simulink model "Main_A"  (R2021a)
settings: Solver=daessc  StartTime=0.0  StopTime=20  RelTol=1e-3
model workspace (MAT data in the model file):
  VEH.Mass = 1181
  VEH.StaticNormalFrontLoad.FR = 264.666666667
  VEH.StaticNormalFrontLoad.FL = 264.666666667
  VEH.StaticNormalRearLoad.RR = 322
  VEH.StaticNormalRearLoad.RL = 322
  VEH.WheelBase = 3.075
  VEH.FrontAxlePositionfromCG = 1.515
  VEH.RearAxlePositionfromCG = 1.504
  VEH.HeightCG = 0.134
  VEH.FrontalArea = 2.11
  VEH.DragCoefficient = 0.33
  VEH.NumberOfWheelsPerAxle = 2
  VEH.PitchMomentInertia = 1922.66666667
  VEH.RollMomentInertia = 432.333333333
  VEH.YawMomentInertia = 2066
  VEH.SteeringRatio = 18
  VEH.TrackWidth = 1.922
  VEH.SprungMass = 1096.72266667
  VEH.InitialLongPosition = -118
  VEH.InitialLatPosition = 3.125
  VEH.InitialVertPosition = 0
  VEH.InitialRollAngle = 0
  VEH.InitialPitchAngle = 0
  VEH.InitialYawAngle = 0
  VEH.InitialLongVel = 0
  VEH.InitialLatVel = 0
  VEH.InitialVertVel = 0
  VEH.InitialRollRate = 0
  VEH.InitialPitchRate = 0
  VEH.InitialYawRate = 0
undefined symbols (not defined in the file): dT, Mu, MuSplit, P_ABSPressureRateMax, P_BrakePressureMax, P_PedalTravelRateMax, P_RefLine4SplitMue, P_RefLine_On, P_RefLineIsX, P_SplitMu_On, P_SplitMuOnlyAtBraking, P_SteeringMax, P_TorqueMax, t_Brake
libraries: sim3dlib x2, simulink_extras x1, vehdynlibsteering x1, sim3dautolib x1, simulink x1, vehdynlibviscommon x1
(part 1 of 2)
settings Model: OrderedModelArguments=off  Creator=Farid  LastModifiedBy=aguil
settings SolverCC: AlgebraicLoopSolver=TrustRegion
settings DebuggingCC: SFMachineParentedDataDiag=warning

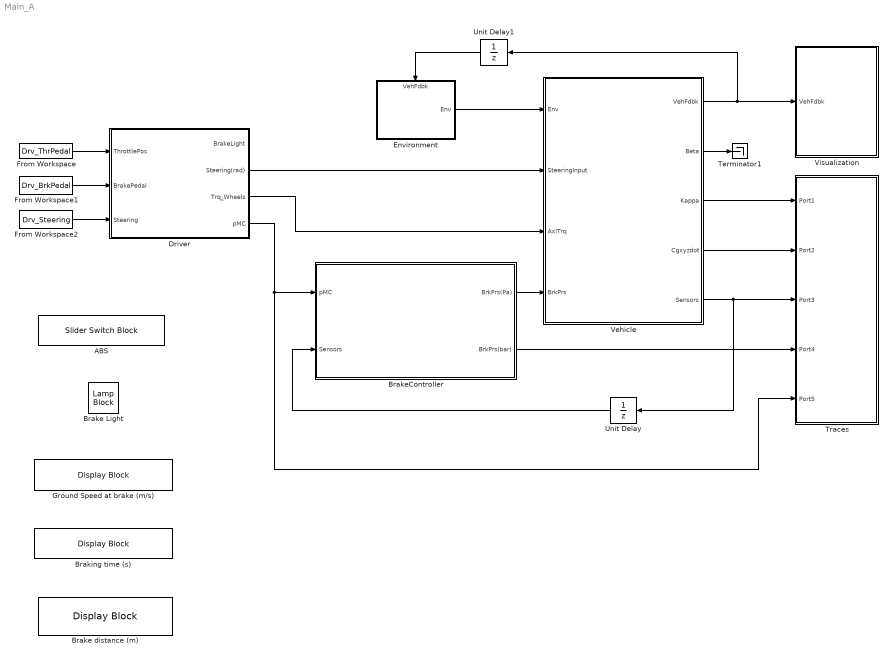
== system Main_A ==
  ABS : SliderSwitchBlock  LabelPosition=Hide
      settings: Values={{'Off', 'On'}, [0 1]}
  Brake Light : LampBlock  LabelPosition=Hide
  Brake distance (m) : DisplayBlock  LabelPosition=Hide  Format=short  Transparency=1
  BrakeController : Subsystem
      mask Display: image('ESP.jpg'); % Use "Edit Image" on toolstrip to change.
  Braking time (s) : DisplayBlock  LabelPosition=Hide  Format=short  Transparency=1
  Driver : Subsystem
  Environment : Subsystem
      settings: PortSchema="{\"entries\":[{\"content\":{\"sides\":[{\"content\":{\"connectorIds\":[]},\"type\":\"ConnectorPlacement.EquallySpacedRectSide\",\"uuid\":\"db779631-5d12-4b7d-908c-0777e0f771c7\"},{\"content\":{\"connectorIds\":[\"Out1\"],\"side\":\"RIGHT\"},\"type\":\"ConnectorPlacement.EquallySpacedRectSide\",\"uuid\":\"a6ec5440-a008-4eb7-8ac9-30b9ee520514\"},{\"content\":{\"connectorIds\":[\"In1\"],\"side\":\"TOP\"},\"type\":\"ConnectorPlacement.EquallySpacedRectSide\",\"uuid\":\"a69fe3ec-df71-47d6-bb93-a6977ac564e9\"},{\"content\":{\"connectorIds\":[],\"side\":\"HIDDEN\"},\"type\":\"ConnectorPlacement.EquallySpacedRectSide\",\"uuid\":\"922b3558-1bf2-4b3b-9005-bb850a1f68da\"}]},\"type\":\"ConnectorPlacement.EquallySpacedConnector\",\"uuid\":\"4d8e08d4-b256-4397-9456-a3bf1aeb88e0\"}],\"packageUris\":[\"http://schema.mathworks.com/mf0/Connector/R2020b\"],\"version\":\"1.0\"}"
  From Workspace : FromWorkspace  VariableName=Drv_ThrPedal  SampleTime=dT
  From Workspace1 : FromWorkspace  VariableName=Drv_BrkPedal  SampleTime=dT
  From Workspace2 : FromWorkspace  VariableName=Drv_Steering  SampleTime=dT
  Ground Speed at brake (m/s) : DisplayBlock  LabelPosition=Hide  Format=short  Transparency=1
  Terminator1 : Terminator
  Traces : Subsystem
  Unit Delay : UnitDelay  SampleTime=-1  HasFrameUpgradeWarning=on
  Unit Delay1 : UnitDelay  SampleTime=-1  HasFrameUpgradeWarning=on
  Vehicle : Subsystem
  Visualization : Subsystem
  wires:
  From Workspace/1 -> Driver/1(ThrottlePos)
  Driver/4(pMC) -> Traces/5(Port5), BrakeController/1(pMC)
  From Workspace1/1 -> Driver/2(BrakePedal)
  Driver/2(Steering(rad)) -> Vehicle/2(SteeringInput)
  Driver/3(Trq_Wheels) -> Vehicle/3(AxlTrq)
  BrakeController/1(BrkPrs(Pa)) -> Vehicle/4(BrkPrs)
  Environment/1(Env) -> Vehicle/1(Env)
  Vehicle/1(VehFdbk) -> Unit Delay1/1, Visualization/1(VehFdbk)
  Vehicle/5(Sensors) -> Unit Delay/1, Traces/3(Port3)
  Unit Delay/1 -> BrakeController/2(Sensors)
  BrakeController/2(BrkPrs(bar)) -> Traces/4(Port4)
  Vehicle/2(Beta) -> Terminator1/1
  Vehicle/3(Kappa) -> Traces/1(Port1)
  Vehicle/4(Cgxyzdot) -> Traces/2(Port2)
  From Workspace2/1 -> Driver/3(Steering)
  Unit Delay1/1 -> Environment/1(VehFdbk)

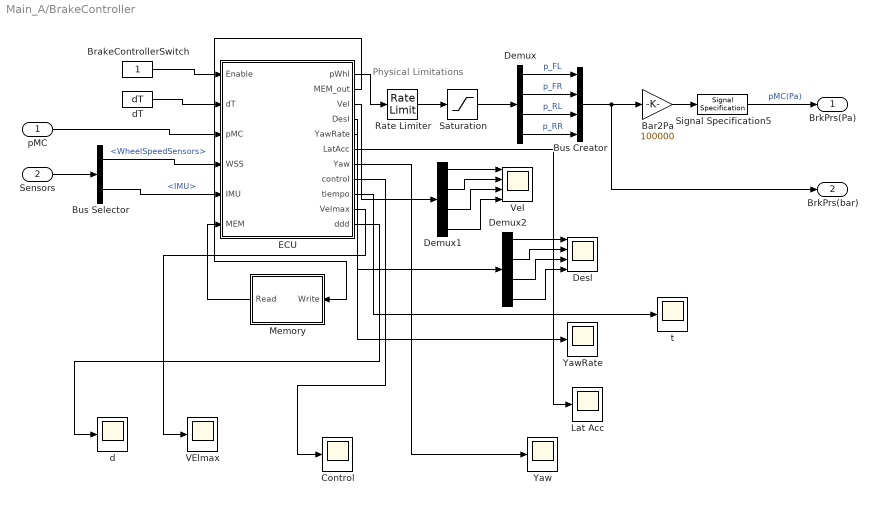
== system Main_A/BrakeController ==
  note: Physical Limitations
  pMC : Inport
  Sensors : Inport  Port=2
  Bar2Pa : Gain  Gain=100000
  BrakeControllerSwitch : Constant
  Bus Creator : BusCreator  Inputs=4
  Bus Selector : BusSelector  OutputSignals=WheelSpeedSensors,IMU
  Control : Scope
  Demux : Demux
  Demux1 : Demux
  Demux2 : Demux
  Desl : Scope  NumInputPorts=4
  ECU : MATLAB Function  TreatAsAtomicUnit=on
  Lat Acc : Scope
  Memory : Subsystem
  Rate Limiter : RateLimiter  RisingSlewLimit=P_ABSPressureRateMax  FallingSlewLimit=-P_ABSPressureRateMax  SampleTimeMode=inherited
  Saturation : Saturate  UpperLimit=P_BrakePressureMax  LowerLimit=0
  Signal Specification5 : SignalSpecification  Unit=Pa
  VElmax : Scope
  Vel : Scope  NumInputPorts=4
  Yaw : Scope
  YawRate : Scope
  d : Scope
  dT : Constant  Value=dT
  t : Scope
  BrkPrs(Pa) : Outport
  BrkPrs(bar) : Outport  Port=2
  wires:
  Demux/1 -> Bus Creator/1  "p_FL"
  Demux/2 -> Bus Creator/2  "p_FR"
  Demux/3 -> Bus Creator/3  "p_RL"
  Demux/4 -> Bus Creator/4  "p_RR"
  Bus Creator/1 -> BrkPrs(bar)/1, Bar2Pa/1
  Bar2Pa/1 -> Signal Specification5/1
  Signal Specification5/1 -> BrkPrs(Pa)/1  "pMC(Pa)"
  ECU/1(pWhl) -> Rate Limiter/1
  Bus Selector/1 -> ECU/4(WSS)  "<WheelSpeedSensors>"
  Bus Selector/2 -> ECU/5(IMU)  "<IMU>"
  Sensors/1 -> Bus Selector/1
  dT/1 -> ECU/2(dT)
  Rate Limiter/1 -> Saturation/1
  pMC/1 -> ECU/3(pMC)
  Saturation/1 -> Demux/1
  BrakeControllerSwitch/1 -> ECU/1(Enable)
  ECU/2(MEM_out) -> Memory/1(Write)
  Memory/1(Read) -> ECU/6(MEM)
  ECU/3(Vel) -> Demux1/1
  Demux1/1 -> Vel/1
  Demux1/2 -> Vel/2
  Demux1/3 -> Vel/3
  Demux1/4 -> Vel/4
  Demux2/2 -> Desl/2
  Demux2/4 -> Desl/4
  Demux2/1 -> Desl/1
  Demux2/3 -> Desl/3
  ECU/4(Desl) -> Demux2/1
  ECU/5(YawRate) -> YawRate/1
  ECU/6(LatAcc) -> Lat Acc/1
  ECU/7(Yaw) -> Yaw/1
  ECU/8(control) -> Control/1
  ECU/9(tiempo) -> t/1
  ECU/10(Velmax) -> VElmax/1
  ECU/11(ddd) -> d/1

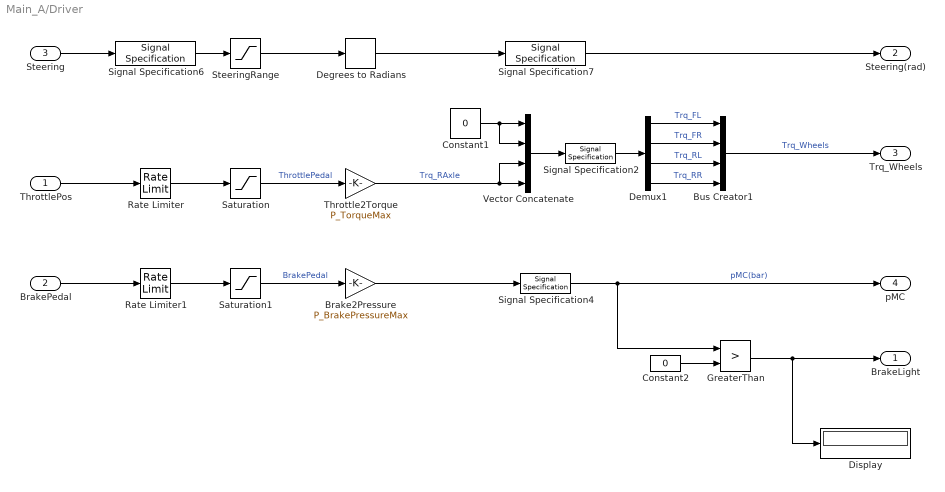
== system Main_A/Driver ==
  ThrottlePos : Inport
  BrakePedal : Inport  Port=2
  Steering : Inport  Port=3
  Brake2Pressure : Gain  Gain=P_BrakePressureMax
  Bus Creator1 : BusCreator  Inputs=4
  Constant1 : Constant  Value=0
  Constant2 : Constant  Value=0
  Degrees to Radians : simulink_extras/Transformations/Degrees to Radians
  Demux1 : Demux
  Display : Display
  GreaterThan : RelationalOperator  Operator=>  OutDataTypeStr=boolean  RndMeth=Simplest
  Rate Limiter : RateLimiter  RisingSlewLimit=P_PedalTravelRateMax  FallingSlewLimit=-P_PedalTravelRateMax  SampleTimeMode=inherited
  Rate Limiter1 : RateLimiter  RisingSlewLimit=P_PedalTravelRateMax  FallingSlewLimit=-P_PedalTravelRateMax  SampleTimeMode=inherited
  Saturation : Saturate  UpperLimit=1  LowerLimit=0
  Saturation1 : Saturate  UpperLimit=1  LowerLimit=0
  Signal Specification2 : SignalSpecification  Unit=N*m
  Signal Specification4 : SignalSpecification  Unit=bar
  Signal Specification6 : SignalSpecification  Unit=deg
  Signal Specification7 : SignalSpecification  Unit=rad
  SteeringRange : Saturate  UpperLimit=P_SteeringMax  LowerLimit=-P_SteeringMax
  Throttle2Torque : Gain  Gain=P_TorqueMax
  Vector Concatenate : Concatenate  NumInputs=4
  BrakeLight : Outport
  Steering(rad) : Outport  Port=2
  Trq_Wheels : Outport  Port=3
  pMC : Outport  Port=4
  wires:
  Brake2Pressure/1 -> Signal Specification4/1
  Constant1/1 -> Vector Concatenate/2, Vector Concatenate/1
  SteeringRange/1 -> Degrees to Radians/1
  Demux1/3 -> Bus Creator1/3  "Trq_RL"
  Degrees to Radians/1 -> Signal Specification7/1
  Demux1/2 -> Bus Creator1/2  "Trq_FR"
  ThrottlePos/1 -> Rate Limiter/1
  Signal Specification4/1 -> pMC/1, GreaterThan/1  "pMC(bar)"
  Demux1/1 -> Bus Creator1/1  "Trq_FL"
  Saturation1/1 -> Brake2Pressure/1  "BrakePedal"
  Bus Creator1/1 -> Trq_Wheels/1  "Trq_Wheels"
  Throttle2Torque/1 -> Vector Concatenate/3, Vector Concatenate/4  "Trq_RAxle"
  Steering/1 -> Signal Specification6/1
  Signal Specification6/1 -> SteeringRange/1
  Demux1/4 -> Bus Creator1/4  "Trq_RR"
  Saturation/1 -> Throttle2Torque/1  "ThrottlePedal"
  BrakePedal/1 -> Rate Limiter1/1
  Rate Limiter1/1 -> Saturation1/1
  Rate Limiter/1 -> Saturation/1
  Signal Specification7/1 -> Steering(rad)/1
  GreaterThan/1 -> Display/1, BrakeLight/1
  Constant2/1 -> GreaterThan/2
  Signal Specification2/1 -> Demux1/1
  Vector Concatenate/1 -> Signal Specification2/1

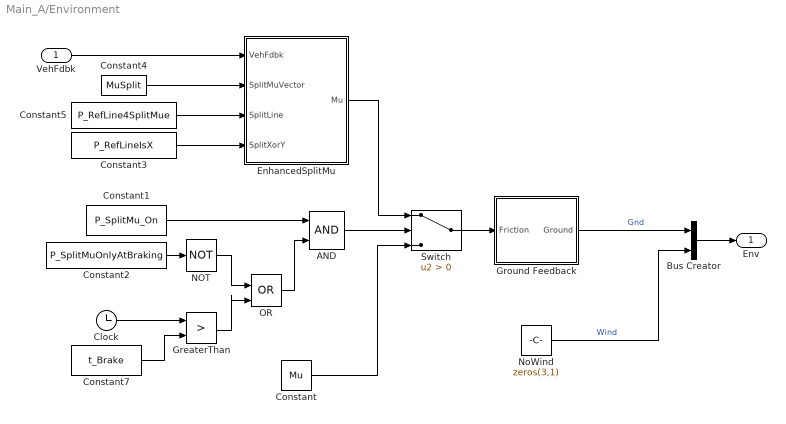
== system Main_A/Environment ==
  VehFdbk : Inport
  AND : Logic  IconShape=distinctive  AllPortsSameDT=off  OutDataTypeStr=boolean
  Bus Creator : BusCreator  Inputs=2
  Clock : Clock
  Constant : Constant  Value=Mu
  Constant1 : Constant  Value=P_SplitMu_On
  Constant2 : Constant  Value=P_SplitMuOnlyAtBraking
  Constant3 : Constant  Value=P_RefLineIsX
  Constant4 : Constant  Value=MuSplit
  Constant5 : Constant  Value=P_RefLine4SplitMue
  Constant7 : Constant  Value=t_Brake
  EnhancedSplitMu : Subsystem
  GreaterThan : RelationalOperator  Operator=>  OutDataTypeStr=boolean  RndMeth=Simplest
  Ground Feedback : Subsystem  Variant=on  VariantControlMode=label  LabelModeActiveChoice=1
  NOT : Logic  Operator=NOT  IconShape=distinctive  AllPortsSameDT=off  OutDataTypeStr=boolean
  NoWind : Constant  Value=zeros(3,1)
  OR : Logic  Operator=OR  IconShape=distinctive  AllPortsSameDT=off  OutDataTypeStr=boolean
  Switch : Switch  Criteria=u2 > Threshold
  Env : Outport
  wires:
  NoWind/1 -> Bus Creator/2  "Wind"
  Bus Creator/1 -> Env/1
  Clock/1 -> GreaterThan/1
  Constant7/1 -> GreaterThan/2
  Ground Feedback/1(Ground) -> Bus Creator/1  "Gnd"
  Switch/1 -> Ground Feedback/1(Friction)
  Constant/1 -> Switch/3
  VehFdbk/1 -> EnhancedSplitMu/1(VehFdbk)
  Constant4/1 -> EnhancedSplitMu/2(SplitMuVector)
  Constant5/1 -> EnhancedSplitMu/3(SplitLine)
  EnhancedSplitMu/1(Mu) -> Switch/1
  AND/1 -> Switch/2
  Constant1/1 -> AND/1
  OR/1 -> AND/2
  GreaterThan/1 -> OR/2
  Constant2/1 -> NOT/1
  NOT/1 -> OR/1
  Constant3/1 -> EnhancedSplitMu/4(SplitXorY)

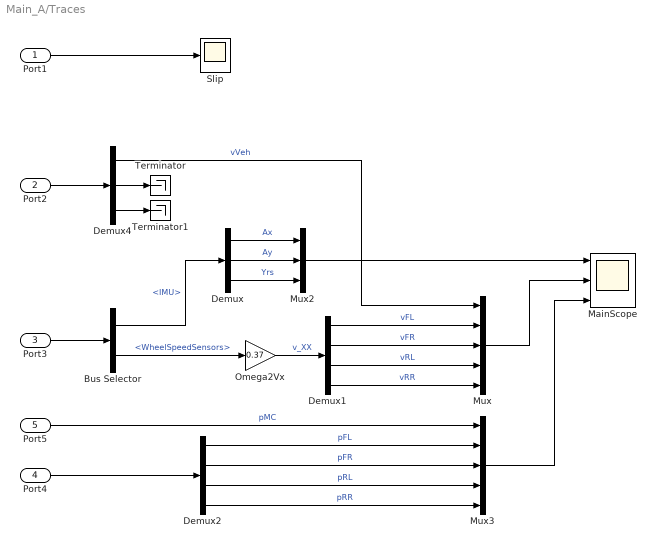
== system Main_A/Traces ==
  Port1 : Inport
  Port2 : Inport  Port=2
  Port3 : Inport  Port=3
  Port4 : Inport  Port=4
  Port5 : Inport  Port=5
  Bus Selector : BusSelector  OutputSignals=IMU,WheelSpeedSensors
  Demux : Demux  Outputs=3
  Demux1 : Demux
  Demux2 : Demux
  Demux4 : Demux  Outputs=3
  MainScope : Scope  NumInputPorts=3
  Mux : Mux  Inputs=5
  Mux2 : Mux  Inputs=3
  Mux3 : Mux  Inputs=5
  Omega2Vx : Gain  Gain=0.37
  Slip : Scope
  Terminator : Terminator
  Terminator1 : Terminator
  wires:
  Demux/2 -> Mux2/2  "Ay"
  Port2/1 -> Demux4/1
  Demux4/1 -> Mux/1  "vVeh"
  Demux/3 -> Mux2/3  "Yrs"
  Demux/1 -> Mux2/1  "Ax"
  Port3/1 -> Bus Selector/1
  Port1/1 -> Slip/1
  Demux4/2 -> Terminator/1
  Demux4/3 -> Terminator1/1
  Mux/1 -> MainScope/2
  Port5/1 -> Mux3/1  "pMC"
  Port4/1 -> Demux2/1
  Bus Selector/1 -> Demux/1  "<IMU>"
  Bus Selector/2 -> Omega2Vx/1  "<WheelSpeedSensors>"
  Mux2/1 -> MainScope/1
  Omega2Vx/1 -> Demux1/1  "v_XX"
  Demux1/1 -> Mux/2  "vFL"
  Demux1/2 -> Mux/3  "vFR"
  Demux1/3 -> Mux/4  "vRL"
  Demux1/4 -> Mux/5  "vRR"
  Demux2/1 -> Mux3/2  "pFL"
  Demux2/2 -> Mux3/3  "pFR"
  Demux2/3 -> Mux3/4  "pRL"
  Demux2/4 -> Mux3/5  "pRR"
  Mux3/1 -> MainScope/3

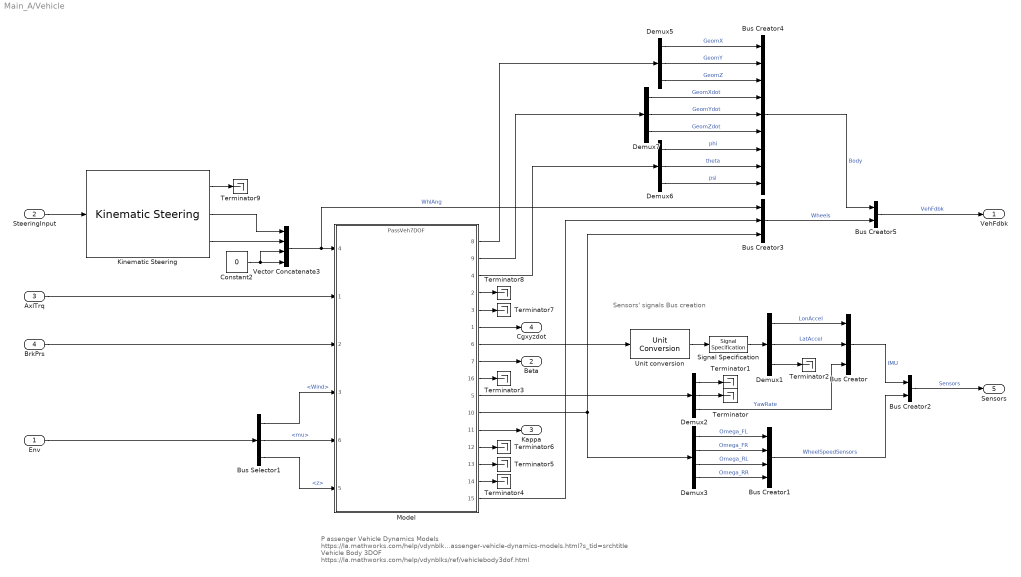
== system Main_A/Vehicle ==
  note: P assenger Vehicle Dynamics Models
      | https://la.mathworks.com/help/vdynblks/ug/passenger-vehicle-dynamics-models.html?s_tid=srchtitle
      | Vehicle Body 3DOF
      | https://la.mathworks.com/help/vdynblks/ref/vehiclebody3dof.html
  note: Sensors' signals Bus creation
  Env : Inport
  SteeringInput : Inport  Port=2
  AxlTrq : Inport  Port=3
  BrkPrs : Inport  Port=4
  Bus Creator : BusCreator  Inputs=3
  Bus Creator1 : BusCreator  Inputs=4
  Bus Creator2 : BusCreator  Inputs=2
  Bus Creator3 : BusCreator  Inputs=3
  Bus Creator4 : BusCreator  Inputs=9
  Bus Creator5 : BusCreator  Inputs=2
  Bus Selector1 : BusSelector  OutputSignals=Wind,Gnd.mu,Gnd.z
  Constant2 : Constant  Value=0
  Demux{1..2,5..7} (5 alike) : Demux  Outputs=3
  Demux3 : Demux
  Kinematic Steering : vehdynlibsteering/Kinematic Steering  StrgType=Ackerman  StrgRatioType=Constant  Loc=Front  NrmlFctr=0.01  TrckWdth=VEH.TrackWidth  WhlBase=VEH.WheelBase  Db=0  StrgRng=P_SteeringMax*pi/180  StrgAngBpts="[-6.2832   -5.0265   -3.7699   -2.5133   -1.2566         0    1.2566    2.5133    3.7699    5.0265    6.2832]"  StrgRatioTbl=|  StrgRatio=P_SteeringRatio  StrgArmLngth=0.1  RckCsLngth=0.5  TieRodLngth=0.248  D=0.2  PnnRadius=0.0057  PnnRadiusTbl="[0.0055    0.0055    0.0056    0.0057    0.0058    0.0057    0.0057    0.0057    0.0056    0.0055    0.0055]"  RodLngth=0.1  ParaArmLngth=0.9  aMode=2
      | [13.5000   13.3750   13.2500   13.1250   13.0000   13.0000   13.0000   13.1250   13.2500   13.3750   13.5000
      | ]
  Model : ModelReference  ModelNameDialog=PassVeh7DOF.slx  SimulationMode=Normal  ModelReferenceVersion=2.14
      settings: PortSchema="{\"entries\":[{\"content\":{\"sides\":[{\"content\":{\"connectorIds\":[\"In4\",\"In1\",\"In2\",\"In3\",\"In6\",\"In5\"]},\"type\":\"ConnectorPlacement.EquallySpacedRectSide\",\"uuid\":\"a5af96ca-5392-45ae-a018-53085440adb3\"},{\"content\":{\"connectorIds\":[\"Out8\",\"Out9\",\"Out4\",\"Out2\",\"Out3\",\"Out1\",\"Out6\",\"Out7\",\"Out16\",\"Out5\",\"Out10\",\"Out11\",\"Out12\",\"Out13\",\"Out14\",\"Out15\"],\"side\":\"RIGHT\"},\"type\":\"ConnectorPlacement.EquallySpacedRectSide\",\"uuid\":\"7efd38ed-5f2f-45a4-b29f-cf848eba49e2\"},{\"content\":{\"connectorIds\":[],\"side\":\"TOP\"},\"type\":\"ConnectorPlacement.EquallySpacedRectSide\",\"uuid\":\"08b428b2-8923-4560-97cc-f07723f31628\"}]},\"type\":\"ConnectorPlacement.EquallySpacedConnector\",\"uuid\":\"5e4c1ab4-766b-4d27-829e-7c1b90f8db53\"}],\"packageUris\":[\"http://schema.mathworks.com/mf0/Connector/19700101\"],\"version\":\"1.0\"}"
  Signal Specification : SignalSpecification  Unit=m/s^2
  Terminator{,1..9} (10 alike) : Terminator
  Unit conversion : UnitConversion
  Vector Concatenate3 : Concatenate  NumInputs=4
  VehFdbk : Outport
  Beta : Outport  Port=2
  Kappa : Outport  Port=3
  Cgxyzdot : Outport  Port=4
  Sensors : Outport  Port=5
  wires:
  Bus Creator1/1 -> Bus Creator2/2  "WheelSpeedSensors"
  Demux5/3 -> Bus Creator4/3  "GeomZ"
  Demux3/3 -> Bus Creator1/3  "Omega_RL"
  Demux2/2 -> Terminator/1
  Bus Selector1/2 -> Model/6  "<mu>"
  Demux3/2 -> Bus Creator1/2  "Omega_FR"
  Demux7/1 -> Bus Creator4/4  "GeomXdot"
  Model/7 -> Beta/1
  Demux6/3 -> Bus Creator4/9  "psi"
  AxlTrq/1 -> Model/1
  Demux5/2 -> Bus Creator4/2  "GeomY"
  Demux6/1 -> Bus Creator4/7  "phi"
  Demux6/2 -> Bus Creator4/8  "theta"
  Model/6 -> Unit conversion/1
  Demux3/4 -> Bus Creator1/4  "Omega_RR"
  Model/1 -> Cgxyzdot/1
  Model/16 -> Terminator3/1
  BrkPrs/1 -> Model/2
  Model/4 -> Demux6/1
  Unit conversion/1 -> Signal Specification/1
  Bus Selector1/1 -> Model/3  "<Wind>"
  Demux1/3 -> Terminator2/1
  Demux3/1 -> Bus Creator1/1  "Omega_FL"
  Demux7/2 -> Bus Creator4/5  "GeomYdot"
  Demux5/1 -> Bus Creator4/1  "GeomX"
  Model/9 -> Demux7/1
  Bus Selector1/3 -> Model/5  "<z>"
  Model/15 -> Bus Creator3/2
  Env/1 -> Bus Selector1/1
  Demux7/3 -> Bus Creator4/6  "GeomZdot"
  Bus Creator5/1 -> VehFdbk/1  "VehFdbk"
  Model/8 -> Demux5/1
  Model/11 -> Kappa/1
  Model/13 -> Terminator5/1
  Model/14 -> Terminator4/1
  Model/12 -> Terminator6/1
  Model/3 -> Terminator7/1
  Model/2 -> Terminator8/1
  Bus Creator/1 -> Bus Creator2/1  "IMU"
  Bus Creator4/1 -> Bus Creator5/1  "Body"
  Bus Creator3/1 -> Bus Creator5/2  "Wheels"
  Constant2/1 -> Vector Concatenate3/4, Vector Concatenate3/3
  Vector Concatenate3/1 -> Bus Creator3/1, Model/4  "WhlAng"
  Kinematic Steering/2 -> Vector Concatenate3/1
  Kinematic Steering/3 -> Vector Concatenate3/2
  SteeringInput/1 -> Kinematic Steering/1
  Bus Creator2/1 -> Sensors/1  "Sensors"
  Model/10 -> Demux3/1, Bus Creator3/3
  Demux1/1 -> Bus Creator/1  "LonAccel"
  Demux1/2 -> Bus Creator/2  "LatAccel"
  Model/5 -> Demux2/1
  Signal Specification/1 -> Demux1/1
  Kinematic Steering/1 -> Terminator9/1
  Demux2/1 -> Terminator1/1
  Demux2/3 -> Bus Creator/3  "YawRate"

== system Main_A/Visualization ==
  note: To enable/disable the XY Plotter, uncomment or comment the "Vehicle XY Plotter", respectively.
  note: To enable/disable the 3D simulation, double click the "3D Engine" block and select the corresponding option.
  VehFdbk : Inport
  3D Engine : Subsystem  Variant=on  VariantControlMode=label  LabelModeActiveChoice=1  mask(3D Engine){engine3D=Enabled, SceneDesc=Straight road, dt3D=.03, defaultPos=Recommended for scene, X_o=-118, Y_o=3.125, Z_o=0, phi_o=0, theta_o=0, psi_o=0}
      mask prompts: engine3D "3D Engine"; SceneDesc "Scene:"; dt3D "Engine frame rate, dt3D [s]:"; X_o "Initial longitudinal position, X_o [m]:"; Y_o "Initial lateral position, Y_o [m]:"; Z_o "Initial vertical position, Z_o [m]:"; phi_o "Initial roll angle, phi_o [rad]:"; theta_o "Initial pitch angle, theta_o [rad]:"; psi_o "Initial yaw angle, psi_o [rad]:"
      mask help: This subsystem contains the interface blocks which permit the display of the vehicle in the 3D virtual environment. Enable it to view the simulation progress, disable it to inhibit the display.
      mask init:
      | switch get_param(gcb,'engine3D')
      |     case 'Disabled'
      |         set_param(gcb,'OverrideUsingVariant','0')
      |         try
      |             set_param([bdroot '/Environment/Ground Feedback'],'OverrideUsingVariant','0')
      |         catch
      |             disp('Warning: No ground feedback sensor not set')
      |         end
      |     case 'Enabled'
      |         set_param(gcb,'OverrideUsingVariant','1')
      |         try
      |             set_param([bdroot '/Environment/Ground Feedback'],'OverrideUsingVariant','1')
      |         catch
      |             disp('Warning: No ground feedback sensor not set')
      |         end
      |     otherwise
      |         set_param(gcb,'OverrideUsingVariant','0')
      | end
      settings: AttributesFormatString=|
      | %<SceneDesc>
      | %<engine3D>
      mask Help: eval('vdynblkshelp(''vdynblks3dengine'')');
      mask TypeOptions engine3D: Enabled | Disabled
      mask Callback engine3D:
      | switch get_param(gcb,'engine3D')
      |     case 'Disabled'
      |         set_param(gcb,'OverrideUsingVariant','0')
      |     case 'Enabled'
      |        set_param(gcb,'OverrideUsingVariant','1')
      |     otherwise
      |        set_param(gcb,'OverrideUsingVariant','0')
      | end
      mask TypeOptions SceneDesc: 3D Engine/Simulation 3D Scene Configuration/SceneDesc
      mask Callback SceneDesc:
      | defaultStatus = get_param(gcb,'defaultPos');
      | if strcmp(defaultStatus,'Recommended for scene')
      | sceneType = get_param(gcb,'SceneDesc');
      | switch sceneType
      |     case 'Straight road'
      |         set_param(gcb,'X_o', '-118')
      |         set_param(gcb,'Y_o', '3.125')
      |         set_param(gcb,'Z_o', '0')
      |         set_param(gcb,'phi_o', '0')
      |         set_param(gcb,'theta_o', '0')
      |         set_param(gcb,'psi_o', '0')
      |     case 'Curved road'
      |         set_param(gcb,'X_o', '0.2')
      |         set_param(gcb,'Y_o', '-1605.0')
      |         set_param(gcb,'Z_o', '0')
      |         set_param(gcb,'phi_o', '0')
      |         set_param(gcb,'theta_o', '0')
      |         set_param(gcb,'psi_o', '-156*pi/180')
      |     case 'Parking lot'
      |         set_param(gcb,'X_o', '-104.0')
      |         set_param(gcb,'Y_o', '-9.7')
      |         set_param(gcb,'Z_o', '0')
      |         set_param(gcb,'phi_o', '0')
      |         set_param(gcb,'theta_o', '0')
      |         set_param(gcb,'psi_o', '0')
      |     case 'Double lane change'
      |         set_param(gcb,'X_o', '0')
      |         set_param(gcb,'Y_o', '3.125')
      |         set_param(gcb,'Z_o', '0')
      |         set_param(gcb,'phi_o', '0')
      |         set_param(gcb,'theta_o', '0')
      |         set_param(gcb,'psi_o', '0')
      |     case 'Open surface'
      |         set_param(gcb,'X_o', '0')
      |         set_param(gcb,'Y_o', '0')
      |         set_param(gcb,'Z_o', '0')
      |         set_param(gcb,'phi_o', '0')
      |         set_param(gcb,'theta_o', '0')
      |         set_param(gcb,'psi_o', '0')
      |     case 'US highway'
      |         set_param(gcb,'X_o', '3592.00')
      |         set_param(gcb,'Y_o', '2617.00')
      |         set_param(gcb,'Z_o', '-1.0')
      |         set_param(gcb,'phi_o', '0')
      |         set_param(gcb,'theta_o', '0')
      |         set_param(gcb,'psi_o', '0')
      |     case 'US city block'
      |         set_param(gcb,'X_o', '-125.19')
      |         set_param(gcb,'Y_o', '1.65')
      |         set_param(gcb,'Z_o', '-0.04')
      |         set_param(gcb,'phi_o', '0')
      |         set_param(gcb,'theta_o', '0')
      |         set_param(gcb,'psi_o', '0')
      |     case 'Large parking lot'
      |         set_param(gcb,'X_o', '45.0')
      |         set_param(gcb,'Y_o', '54.7')
      |         set_param(gcb,'Z_o', '0.0')
      |         set_param(gcb,'phi_o', '0')
      |         set_param(gcb,'theta_o', '0')
      |         set_param(gcb,'psi_o', '-pi/2')
      |     case 'Virtual Mcity'
      |         set_param(gcb,'X_o', '-26.0')
      |         set_param(gcb,'Y_o', '76.0')
      |         set_param(gcb,'Z_o', '0.0')
      |         set_param(gcb,'phi_o', '0')
      |         set_param(gcb,'theta_o', '0')
      |         set_param(gcb,'psi_o', '-40*pi/180')
      |     otherwise
      |         set_param(gcb,'X_o', '0')
      |         set_param(gcb,'Y_o', '0')
      |         set_param(gcb,'Z_o', '0')
      |         set_param(gcb,'phi_o', '0')
      |         set_param(gcb,'theta_o', '0')
      |         set_param(gcb,'psi_o', '0')
      | end
      | end
      mask TypeOptions defaultPos: Recommended for scene | User-specified
      mask DialogControl engineConfig Prompt: 3D Engine Settings
      mask DialogControl posSetup Prompt: Initial vehicle position
      mask DialogControl posSetupDesc Prompt: To use these initial vehicle positions, first Apply the initial values and then click Update the model workspaces with the initial values.
      mask DialogControl setModelPos Prompt: Update model workspaces with initial values
      mask DialogControl setModelPos Callback:
      | if strcmp(get_param(bdroot(gcb),'SimulationStatus'),'stopped')
      |     sceneType = get_param(gcb,'SceneDesc');
      |     rootModel = bdroot(gcb);
      |     ws = get_param(rootModel, 'modelworkspace');
      |     VEH = getVariable(ws,'VEH');
      |     ParamList={'X_o',[1,1],{};'Y_o',[1,1],{};'Z_o',[1,1],{};'phi_o',[1,1],{'gte',-pi/2;'lte',pi/2};'theta_o',[1,1],{'gte',-pi/2;'lte',pi/2};'psi_o',[1,1],{'gte',-2*pi;'lte',2*pi}};
      |     paramStruct = autoblkscheckparams(gcb, '3D Engine',ParamList);
      |     VEH.InitialLongPosition = paramStruct.X_o;
      |     VEH.InitialLatPosition = paramStruct.Y_o;
      |     VEH.InitialVertPosition = paramStruct.Z_o;
      |     VEH.InitialRollAngle = paramStruct.phi_o;
      |     VEH.InitialPitchAngle = paramStruct.theta_o;
      |     VEH.InitialYawAngle = paramStruct.psi_o;
      |     assignin(ws,'VEH',VEH);
      | %   modelList = {'PassVeh14DOF','PassVeh7DOF'};
      |     modelList = {'PassVeh7DOF'}
      |     for idx =1:length(modelList)
      | %         try
      |             load_system(modelList{idx});
      |             ws = get_param(modelList{idx}, 'modelworkspace');
      |             assignin(ws,'VEH',VEH);
      |             save_system(modelList{idx});
      |             close_system(modelList{idx});
      | %         catch
      | %             disp(['Cannot find ' modelList{idx}])
      | %         end
      |     end
      | end
      mask Display: disp('3D Engine')
  Bus Selector2 : BusSelector  OutputSignals=Body.phi,Body.theta,Body.psi  OutputAsBus=on
  Bus Selector5 : BusSelector  OutputSignals=Wheels.WhlAng  OutputAsBus=on
  Bus Selector6 : BusSelector  OutputSignals=Body.GeomX,Body.GeomY,Body.GeomZ  OutputAsBus=on
  Bus Selector7 : BusSelector  OutputSignals=Body.GeomXdot,Body.GeomYdot,Body.GeomZdot  OutputAsBus=on
  Bus to Vector : BusToVector
  Bus to Vector1 : BusToVector
  Bus to Vector2 : BusToVector
  RefLine : Subsystem
  Vehicle XY Plotter : Subsystem  mask(Vehicle XY Plotter){a=VEH.FrontAxlePositionfromCG, b=VEH.RearAxlePositionfromCG, w=VEH.TrackWidth, figBorder=10, bufferSize=1024, extRef=on, pltDT=0.1}
      mask prompts: a "Distance to front axle from CG, a [m]:"; b "Distance to rear axle from CG, b [m]:"; w "Track width, w [m]:"; figBorder "Distance to figure borders, figBorder [m]:"; bufferSize "Path buffer sampe size, bufferSize []:"; extRef "Plot path reference, extRef"; pltDT "Plot update rate, pltDT [s]:"
      mask help:
      | This block will display a MATLAB figure which indicates the vehicle path, current position and heading velocity.
      | An optional path reference is also provided.
      mask init:
      | if autoblkschecksimstopped(gcb)
      |     PortName = 'RefXYZ';
      |     InportOption  = {'built-in/Ground', [PortName, ' Ground'];...
      |         'built-in/Inport',PortName };
      |     if ~strcmp(get_param(gcb,'extRef'),'on')
      |         NewBlkHdl = autoblksreplaceblock(gcb, InportOption, 1);
      |         set_param(NewBlkHdl, 'ShowName', 'off');
      |     else
      |         autoblksreplaceblock(gcb, InportOption, 2);
      |     end
      | end
      mask TypeOptions a: Vehicle XY Plotter/a
      mask TypeOptions b: Vehicle XY Plotter/b
      mask TypeOptions w: Vehicle XY Plotter/w
      mask TypeOptions figBorder: Vehicle XY Plotter/figBorder
      mask TypeOptions bufferSize: Vehicle XY Plotter/bufferSize
  wires:
  Bus Selector7/1 -> Bus to Vector1/1
  Bus to Vector1/1 -> Vehicle XY Plotter/3(InertXdotYdotZdot)
  Bus to Vector/1 -> Vehicle XY Plotter/1(InertXYZ)
  Bus Selector5/1 -> Vehicle XY Plotter/4(WhlAng)
  Bus to Vector2/1 -> Vehicle XY Plotter/2(InertAng)
  Bus Selector2/1 -> Bus to Vector2/1
  Bus Selector6/1 -> Bus to Vector/1
  RefLine/1(Ref) -> Vehicle XY Plotter/5(RefXYZ)
  VehFdbk/1 -> Bus Selector7/1, Bus Selector6/1, Bus Selector2/1, Bus Selector5/1, 3D Engine/1(VehFdbk)

== system Main_A/BrakeController/Memory ==
  note: The way simulink and the 'MATLAB function' block work does not allow storage of local variables whithin the script/block. Therefore, it was necessary to find a way to pass such variables to the next iteration. This is done by connecting an output port that contains all these variables to an input port that will receive them, and in between those 2 ports it is required to connect a 'Unit Delay', which all it does is: it receives whatever value is sent to it in simulation's time step K, holds it and then in time step K+1 sends it out.
  note: It is recommended that the size of the Memory vector (column vector) is defined by a fixed value, in order to avoid possible compilation errors in case the script inside ECU block does not correctly handles memory allocation. Thus, here it is defined in the 'Unit Delay' block, with a default value of 50. This number means that it is possible to handle up to a 50 local variables in the 'Matlab Function Block' ECU, quite more than enough.
  Write : Inport
  Unit Delay : UnitDelay  InitialCondition=zeros(50,1)  SampleTime=-1  HasFrameUpgradeWarning=on
  Read : Outport
  wires:
  Unit Delay/1 -> Read/1
  Write/1 -> Unit Delay/1

== system Main_A/Environment/EnhancedSplitMu ==
  VehFdbk : Inport
  SplitMuVector : Inport  Port=2  PortDimensions=2
  SplitLine : Inport  Port=3
  SplitXorY : Inport  Port=4
  Bus Selector : BusSelector  OutputSignals=Body.GeomX,Body.GeomY,Body.psi
  Constant1 : Constant  Value=VEH.TrackWidth
  Constant2 : Constant  Value=VEH.FrontAxlePositionfromCG
  Constant3 : Constant  Value=VEH.RearAxlePositionfromCG
  Mux : Mux
  SplitMu Function : MATLAB Function  TreatAsAtomicUnit=on
  Vector Concatenate : Concatenate  NumInputs=3
  Mu : Outport
  wires:
  Bus Selector/1 -> SplitMu Function/2(X)  "<GeomX>"
  Constant3/1 -> Vector Concatenate/3
  Constant2/1 -> Vector Concatenate/2
  SplitMu Function/1(mu_FL) -> Mux/1
  SplitMu Function/4(mu_RR) -> Mux/4
  Vector Concatenate/1 -> SplitMu Function/1(VehDim)
  Bus Selector/3 -> SplitMu Function/4(psi)  "<psi>"
  Constant1/1 -> Vector Concatenate/1
  Bus Selector/2 -> SplitMu Function/3(Y)  "<GeomY>"
  SplitLine/1 -> SplitMu Function/6(SplitLine)
  SplitMu Function/2(mu_FR) -> Mux/2
  SplitMuVector/1 -> SplitMu Function/5(SplitMu)
  SplitMu Function/3(mu_RL) -> Mux/3
  VehFdbk/1 -> Bus Selector/1
  Mux/1 -> Mu/1
  SplitXorY/1 -> SplitMu Function/7(XorY)

== system Main_A/Environment/Ground Feedback ==
  note: 1) Add Subsystem or Model blocks as valid variant choices.
      | 2) You cannot connect blocks at this level. At simulation, connectivity is automatically
      | determined, based on the active variant and port name matching.
  Friction : Inport
  3D Engine : Subsystem  VariantControl=1
  InputBased : Subsystem  VariantControl=0
  Ground : Outport  VectorParamsAs1DForOutWhenUnconnected=off

== system Main_A/Visualization/3D Engine ==
  note: 1) Add Subsystem or Model blocks as valid variant choices.
      | 2) You cannot connect blocks at this level. At simulation, connectivity is automatically
      | determined, based on the active variant and port name matching.
  VehFdbk : Inport
  3D Engine : Subsystem  VariantControl=1
  3D Engine Disabled : Subsystem  VariantControl=0

== system Main_A/Visualization/RefLine ==
  Constant1 : Constant  Value=P_RefLineIsX
  Constant2 : Constant  Value=P_RefLine4SplitMue
  Ground : Ground
  Ground1 : Ground
  Ground2 : Ground
  Mux : Mux  Inputs=3
  Mux1 : Mux  Inputs=3
  OnOff : Constant  Value=P_RefLine_On
  Ramp : simulink/Sources/Ramp  slope=20  start=0  InitialOutput=VEH.InitialLongPosition
  Switch : Switch  Criteria=u2 > Threshold
  Switch1 : Switch  Criteria=u2 > Threshold
  Switch2 : Switch  Criteria=u2 > Threshold
  Ref : Outport
  wires:
  OnOff/1 -> Switch/2, Switch1/2
  Switch1/1 -> Mux1/1, Mux/2  "Y"
  Switch/1 -> Mux1/2, Mux/1  "X"
  Ground1/1 -> Mux1/3, Mux/3  "Z"
  Ground2/1 -> Switch/3
  Constant2/1 -> Switch1/1
  Ground/1 -> Switch1/3
  Ramp/1 -> Switch/1
  Mux1/1 -> Switch2/1  "Ref"
  Switch2/1 -> Ref/1  "Ref"
  Constant1/1 -> Switch2/2
  Mux/1 -> Switch2/3  "Ref"

== system Main_A/Visualization/Vehicle XY Plotter ==
  InertXYZ : Inport
  InertAng : Inport  Port=2
  InertXdotYdotZdot : Inport  Port=3
  WhlAng : Inport  Port=4
  RefXYZ : Inport  Port=5
  Rate Transition{1..5} (5 alike) : RateTransition  Deterministic=off  OutPortSampleTime=pltDT
  Vehicle XY Plotter : vehdynlibviscommon/Vehicle XY Plotter  w=w  a=a  b=b  figBorder=figBorder  bufferSize=bufferSize  extStats=off  extTireF=off
      settings: SourceProductBaseCode=VE
  wires:
  InertAng/1 -> Rate Transition2/1  "InertCGDisp"
  InertXdotYdotZdot/1 -> Rate Transition4/1  "InertCGVel"
  InertXYZ/1 -> Rate Transition1/1  "InertCGDisp"
  WhlAng/1 -> Rate Transition5/1  "WhlAng"
  Rate Transition3/1 -> Vehicle XY Plotter/5
  Rate Transition1/1 -> Vehicle XY Plotter/1
  Rate Transition2/1 -> Vehicle XY Plotter/2
  Rate Transition4/1 -> Vehicle XY Plotter/3
  Rate Transition5/1 -> Vehicle XY Plotter/4
  RefXYZ/1 -> Rate Transition3/1

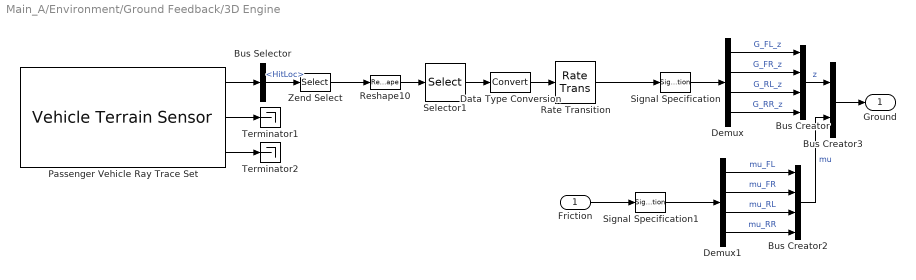
== system Main_A/Environment/Ground Feedback/3D Engine ==
  Friction : Inport
  Bus Creator : BusCreator  Inputs=4
  Bus Creator2 : BusCreator  Inputs=4
  Bus Creator3 : BusCreator  Inputs=2
  Bus Selector : BusSelector  OutputSignals=HitLoc
  Data Type Conversion : DataTypeConversion
  Demux : Demux
  Demux1 : Demux
  Passenger Vehicle Ray Trace Set : sim3dlib/Vehicle Terrain Sensor  Priority=1  ActorTag=SimulinkVehicle1  VehExtEn=Constant  TireRadiiExt=Constant  VehCntrLngthVal=0  TireRadiiVal=0  VehRayLngth=10  LfRayLngth=20  RfRayLngth=20  LrRayLngth=20  RrRayLngth=20  VehRayOffset=0  LfRayOffset=-1  RfRayOffset=-1  LrRayOffset=-1  RrRayOffset=-1  VehEn=on  LfEn=on  RfEn=on  LrEn=on  RrEn=on  DbgEn=off  Ts=.03  aMode=2
      settings: SourceProductBaseCode=DR,UV,VE
  Rate Transition : RateTransition  Integrity=off  Deterministic=off  OutPortSampleTimeOpt=Inherit
  Reshape10 : Reshape  OutputDimensionality=Row vector (2-D)
  Selector1 : Selector  InputPortWidth=5  IndexOptions=Index vector (dialog)  Indices=[2:5]  OutputSizes=1
  Signal Specification : SignalSpecification  Unit=m
  Signal Specification1 : SignalSpecification  Unit=1
  Terminator1 : Terminator
  Terminator2 : Terminator
  Zend Select : Selector  NumberOfDimensions=2  InputPortWidth=3  IndexOptions=Select all,Index vector (dialog)  Indices=[1 3],3  OutputSizes=1,1
  Ground : Outport  VectorParamsAs1DForOutWhenUnconnected=off
  wires:
  Zend Select/1 -> Reshape10/1
  Bus Selector/1 -> Zend Select/1  "<HitLoc>"
  Passenger Vehicle Ray Trace Set/2 -> Terminator1/1
  Passenger Vehicle Ray Trace Set/3 -> Terminator2/1
  Reshape10/1 -> Selector1/1
  Passenger Vehicle Ray Trace Set/1 -> Bus Selector/1
  Selector1/1 -> Data Type Conversion/1
  Demux/2 -> Bus Creator/2  "G_FR_z"
  Demux/1 -> Bus Creator/1  "G_FL_z"
  Demux/4 -> Bus Creator/4  "G_RR_z"
  Demux/3 -> Bus Creator/3  "G_RL_z"
  Signal Specification/1 -> Demux/1
  Signal Specification1/1 -> Demux1/1
  Demux1/1 -> Bus Creator2/1  "mu_FL"
  Bus Creator/1 -> Bus Creator3/1  "z"
  Demux1/3 -> Bus Creator2/3  "mu_RL"
  Demux1/4 -> Bus Creator2/4  "mu_RR"
  Demux1/2 -> Bus Creator2/2  "mu_FR"
  Bus Creator2/1 -> Bus Creator3/2  "mu"
  Bus Creator3/1 -> Ground/1
  Friction/1 -> Signal Specification1/1
  Data Type Conversion/1 -> Rate Transition/1
  Rate Transition/1 -> Signal Specification/1

== system Main_A/Environment/Ground Feedback/InputBased ==
  Friction : Inport
  Bus Creator : BusCreator  Inputs=4
  Bus Creator2 : BusCreator  Inputs=4
  Bus Creator3 : BusCreator  Inputs=2
  Constant1 : Constant  Value=zeros(4,1)
  Demux : Demux
  Demux1 : Demux
  Signal Specification : SignalSpecification  Unit=m
  Signal Specification1 : SignalSpecification  Unit=1
  Ground : Outport  VectorParamsAs1DForOutWhenUnconnected=off
  wires:
  Constant1/1 -> Signal Specification/1
  Signal Specification/1 -> Demux/1
  Demux/4 -> Bus Creator/4  "G_RR_z"
  Demux/1 -> Bus Creator/1  "G_FL_z"
  Demux/3 -> Bus Creator/3  "G_RL_z"
  Demux/2 -> Bus Creator/2  "G_FR_z"
  Bus Creator/1 -> Bus Creator3/1  "z"
  Demux1/3 -> Bus Creator2/3  "mu_RL"
  Demux1/4 -> Bus Creator2/4  "mu_RR"
  Demux1/1 -> Bus Creator2/1  "mu_FL"
  Demux1/2 -> Bus Creator2/2  "mu_FR"
  Bus Creator2/1 -> Bus Creator3/2  "mu"
  Friction/1 -> Signal Specification1/1
  Signal Specification1/1 -> Demux1/1
  Bus Creator3/1 -> Ground/1

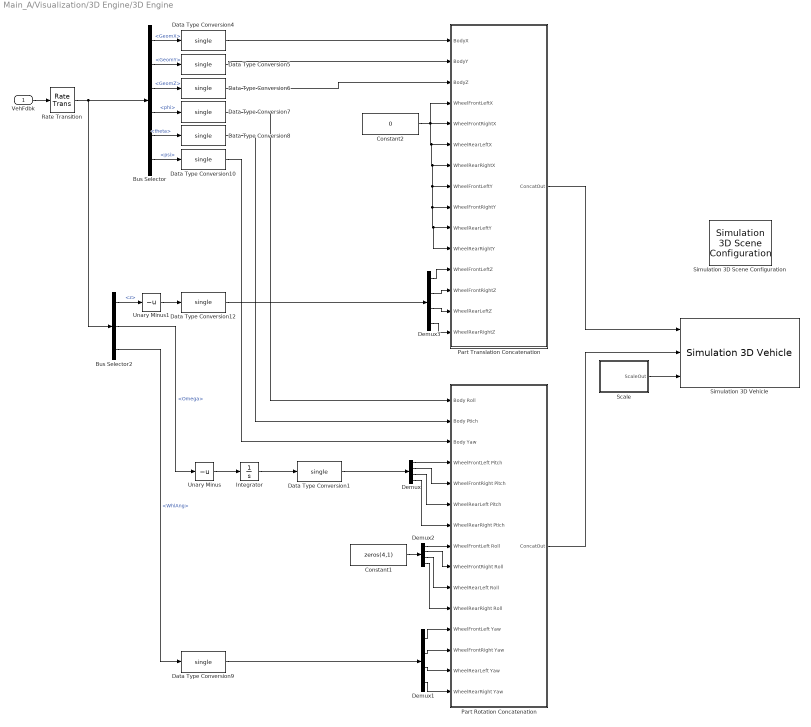
== system Main_A/Visualization/3D Engine/3D Engine ==
  VehFdbk : Inport
  Bus Selector : BusSelector  OutputSignals=Body.GeomX,Body.GeomY,Body.GeomZ,Body.phi,Body.theta,Body.psi
  Bus Selector2 : BusSelector  OutputSignals=Wheels.z,Wheels.Omega,Wheels.WhlAng
  Constant1 : Constant  Value=zeros(4,1)  OutDataTypeStr=single
  Constant2 : Constant  Value=0  OutDataTypeStr=single
  Data Type Conversion{1,4..10,12} (9 alike) : DataTypeConversion  OutDataTypeStr=single
  Demux{,1..3} (4 alike) : Demux
  Integrator : Integrator  WrapState=on  WrappedStateUpperValue=2*pi  WrappedStateLowerValue=0  ZeroCross=off
  Part Rotation Concatenation : Subsystem
  Part Translation Concatenation : Subsystem
  Rate Transition : RateTransition  OutPortSampleTime=dt3D
  Scale : Subsystem
  Simulation 3D Scene Configuration : sim3dlib/Simulation 3D Scene Configuration  Priority=0  ProjectFormat=Default Scenes  SceneDesc=Straight road  ProjectName=C:\Program Files\MATLAB\R2021a\toolbox\shared\sim3d_projects\automotive_project\UE4\WindowsNoEditor\VehicleSimulation.exe  ScenePath=/Game/Maps/HwStrght  vehTagList={'Scene Origin';'SimulinkVehicle1'}  vehTag=SimulinkVehicle1  OpVisEn=off  Ts=dt3D  EnableWindow=on  EnableWeather=off  SunAltitude=40.0  SunAzimuth=90  clouds=10  wind=1  fog=0  rain=0  sensorTag=MainCamera1  sensorId=1  sensorName=MainCamera1  mountLoc=Origin  offsetFlag=off  tmountOffset=[0, 0, 0]  rmountOffset=[0, 0, 0]  HorizontalResolution=1280  VerticalResolution=720  HorizontalFOV=60  mountPoint=[0 0 0]  mountOrientation=[0 0 0]  aMode=aMode  ID=1
      settings: SourceProductBaseCode=DR,UV,VE
  Simulation 3D Vehicle : sim3dautolib/Simulation 3D Vehicle  Priority=-1  PassVehMesh=Muscle car  MeshPath=/MathWorksSimulation/Vehicles/Muscle/Meshes/SK_MuscleCar.SK_MuscleCar  VehColor=Orange  ActorName=SimulinkVehicle1  VehLightsControl=off  HeadlightColor=[ 1, 1, 1 ]  HighBeamIntensity=100000  LowBeamIntensity=60000  HighBeamConeAngle=1.22  LowBeamConeAngle=1.22  LeftHeadlightOrientation=[ 0, 0 ]  RightHeadlightOrientation=[ 0, 0 ]  BrakelightIntensity=500  ReverselightIntensity=500  SignallightIntensity=500  SignallightPeriod=1  SignalPulseWidth=50  Translation=[VEH.InitialLongPosition VEH.InitialLatPosition -VEH.InitialVertPosition; 0 0 0; 0 0 0; 0 0 0; 0 0 0]  Rotation=[VEH.InitialRollAngle VEH.InitialPitchAngle VEH.InitialYawAngle; 0 0 0; 0 0 0; 0 0 0; 0 0 0]  Scale=ones( 5, 3 )  SampleTime=dt3D  ActorType=SimulinkVehicle  ID=1  aMode=2  ActorTag=SimulinkVehicle1
      settings: SourceProductBaseCode=DR,UV,VE
  Unary Minus : UnaryMinus
  Unary Minus1 : UnaryMinus
  wires:
  Unary Minus/1 -> Integrator/1
  Bus Selector2/1 -> Unary Minus1/1  "<z>"
  Rate Transition/1 -> Bus Selector/1, Bus Selector2/1
  Scale/1(ScaleOut) -> Simulation 3D Vehicle/3
  Demux/4 -> Part Rotation Concatenation/7(WheelRearRight Ptich)
  Demux/3 -> Part Rotation Concatenation/6(WheelRearLeft Pitch)
  Demux/2 -> Part Rotation Concatenation/5(WheelFrontRight Pitch)
  Demux/1 -> Part Rotation Concatenation/4(WheelFrontLeft Pitch)
  Constant1/1 -> Demux2/1
  Bus Selector/4 -> Data Type Conversion7/1  "<phi>"
  Part Rotation Concatenation/1(ConcatOut) -> Simulation 3D Vehicle/2
  Part Translation Concatenation/1(ConcatOut) -> Simulation 3D Vehicle/1
  Data Type Conversion12/1 -> Demux3/1
  Demux3/4 -> Part Translation Concatenation/15(WheelRearRightZ)
  Demux3/3 -> Part Translation Concatenation/14(WheelRearLeftZ)
  Demux3/1 -> Part Translation Concatenation/12(WheelFrontLeftZ)
  Demux3/2 -> Part Translation Concatenation/13(WheelFrontRightZ)
  VehFdbk/1 -> Rate Transition/1
  Data Type Conversion6/1 -> Part Translation Concatenation/3(BodyZ)
  Demux1/4 -> Part Rotation Concatenation/15(WheelRearRight Yaw)
  Demux1/3 -> Part Rotation Concatenation/14(WheelRearLeft Yaw)
  Demux2/1 -> Part Rotation Concatenation/8(WheelFrontLeft Roll)
  Demux2/2 -> Part Rotation Concatenation/9(WheelFrontRight Roll)
  Demux2/3 -> Part Rotation Concatenation/10(WheelRearLeft Roll)
  Demux2/4 -> Part Rotation Concatenation/11(WheelRearRight Roll)
  Bus Selector2/3 -> Data Type Conversion9/1  "<WhlAng>"
  Bus Selector2/2 -> Unary Minus/1  "<Omega>"
  Data Type Conversion9/1 -> Demux1/1
  Demux1/1 -> Part Rotation Concatenation/12(WheelFrontLeft Yaw)
  Demux1/2 -> Part Rotation Concatenation/13(WheelFrontRight Yaw)
  Integrator/1 -> Data Type Conversion1/1
  Data Type Conversion1/1 -> Demux/1
  Data Type Conversion8/1 -> Part Rotation Concatenation/2(Body Ptich)
  Data Type Conversion5/1 -> Part Translation Concatenation/2(BodyY)
  Data Type Conversion10/1 -> Part Rotation Concatenation/3(Body Yaw)
  Constant2/1 -> Part Translation Concatenation/5(WheelFrontRightX), Part Translation Concatenation/6(WheelRearLeftX), Part Translation Concatenation/7(WheelRearRightX), Part Translation Concatenation/8(WheelFrontLeftY), Part Translation Concatenation/9(WheelFrontRightY), Part Translation Concatenation/10(WheelRearLeftY), Part Translation Concatenation/11(WheelRearRightY), Part Translation Concatenation/4(WheelFrontLeftX)
  Data Type Conversion4/1 -> Part Translation Concatenation/1(BodyX)
  Data Type Conversion7/1 -> Part Rotation Concatenation/1(Body Roll)
  Bus Selector/1 -> Data Type Conversion4/1  "<GeomX>"
  Bus Selector/2 -> Data Type Conversion5/1  "<GeomY>"
  Bus Selector/3 -> Data Type Conversion6/1  "<GeomZ>"
  Bus Selector/6 -> Data Type Conversion10/1  "<psi>"
  Bus Selector/5 -> Data Type Conversion8/1  "<theta>"
  Unary Minus1/1 -> Data Type Conversion12/1

== system Main_A/Visualization/3D Engine/3D Engine Disabled ==
  VehFdbk : Inport
  Terminator : Terminator
  wires:
  VehFdbk/1 -> Terminator/1

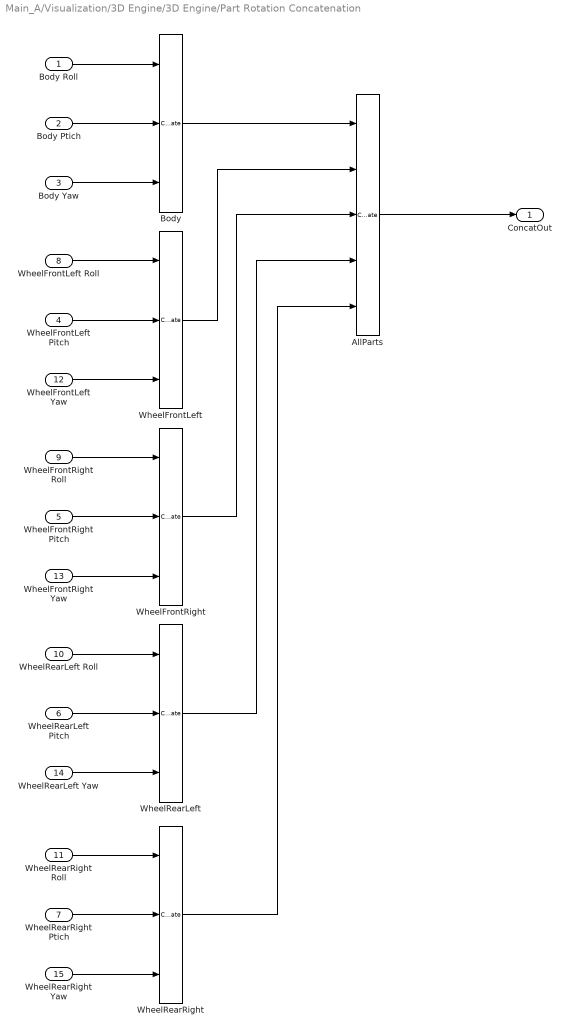
== system Main_A/Visualization/3D Engine/3D Engine/Part Rotation Concatenation ==
  Body Roll : Inport
  Body Ptich : Inport  Port=2
  Body Yaw : Inport  Port=3
  WheelFrontLeft Pitch : Inport  Port=4
  WheelFrontRight Pitch : Inport  Port=5
  WheelRearLeft Pitch : Inport  Port=6
  WheelRearRight Ptich : Inport  Port=7
  WheelFrontLeft Roll : Inport  Port=8
  WheelFrontRight Roll : Inport  Port=9
  WheelRearLeft Roll : Inport  Port=10
  WheelRearRight Roll : Inport  Port=11
  WheelFrontLeft Yaw : Inport  Port=12
  WheelFrontRight Yaw : Inport  Port=13
  WheelRearLeft Yaw : Inport  Port=14
  WheelRearRight Yaw : Inport  Port=15
  AllParts : Concatenate  NumInputs=5  Mode=Multidimensional array
  Body : Concatenate  NumInputs=3  Mode=Multidimensional array  ConcatenateDimension=2
  WheelFrontLeft : Concatenate  NumInputs=3  Mode=Multidimensional array  ConcatenateDimension=2
  WheelFrontRight : Concatenate  NumInputs=3  Mode=Multidimensional array  ConcatenateDimension=2
  WheelRearLeft : Concatenate  NumInputs=3  Mode=Multidimensional array  ConcatenateDimension=2
  WheelRearRight : Concatenate  NumInputs=3  Mode=Multidimensional array  ConcatenateDimension=2
  ConcatOut : Outport  VectorParamsAs1DForOutWhenUnconnected=off
  wires:
  Body Yaw/1 -> Body/3
  WheelFrontLeft Yaw/1 -> WheelFrontLeft/3
  WheelFrontLeft/1 -> AllParts/2
  Body/1 -> AllParts/1
  WheelRearLeft/1 -> AllParts/4
  WheelFrontRight/1 -> AllParts/3
  WheelRearRight Yaw/1 -> WheelRearRight/3
  WheelRearLeft Yaw/1 -> WheelRearLeft/3
  AllParts/1 -> ConcatOut/1
  WheelRearRight/1 -> AllParts/5
  WheelFrontRight Yaw/1 -> WheelFrontRight/3
  Body Roll/1 -> Body/1
  Body Ptich/1 -> Body/2
  WheelFrontLeft Pitch/1 -> WheelFrontLeft/2
  WheelFrontLeft Roll/1 -> WheelFrontLeft/1
  WheelFrontRight Roll/1 -> WheelFrontRight/1
  WheelFrontRight Pitch/1 -> WheelFrontRight/2
  WheelRearLeft Roll/1 -> WheelRearLeft/1
  WheelRearLeft Pitch/1 -> WheelRearLeft/2
  WheelRearRight Roll/1 -> WheelRearRight/1
  WheelRearRight Ptich/1 -> WheelRearRight/2

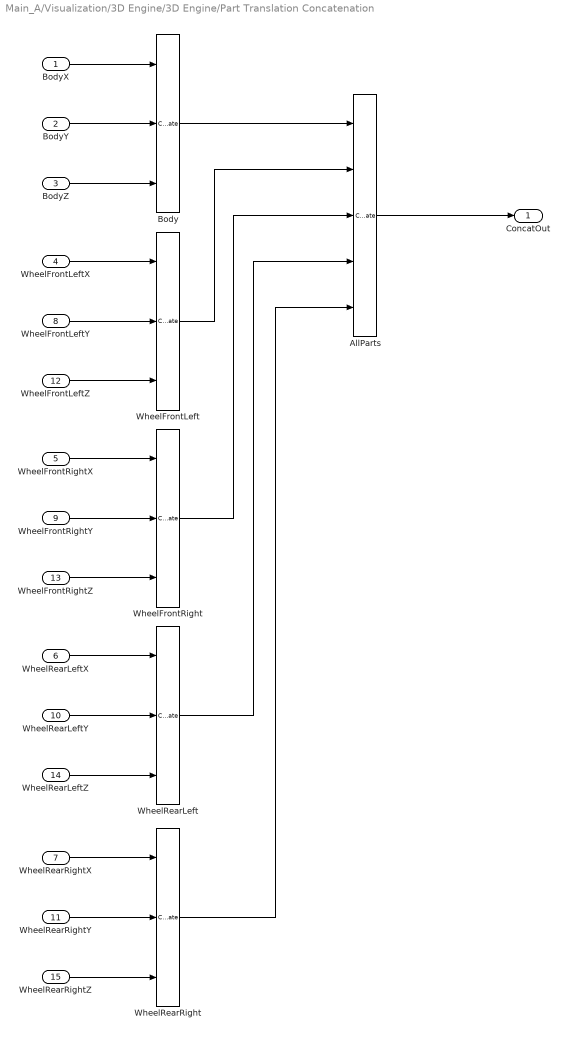
== system Main_A/Visualization/3D Engine/3D Engine/Part Translation Concatenation ==
  BodyX : Inport
  BodyY : Inport  Port=2
  BodyZ : Inport  Port=3
  WheelFrontLeftX : Inport  Port=4
  WheelFrontRightX : Inport  Port=5
  WheelRearLeftX : Inport  Port=6
  WheelRearRightX : Inport  Port=7
  WheelFrontLeftY : Inport  Port=8
  WheelFrontRightY : Inport  Port=9
  WheelRearLeftY : Inport  Port=10
  WheelRearRightY : Inport  Port=11
  WheelFrontLeftZ : Inport  Port=12
  WheelFrontRightZ : Inport  Port=13
  WheelRearLeftZ : Inport  Port=14
  WheelRearRightZ : Inport  Port=15
  AllParts : Concatenate  NumInputs=5  Mode=Multidimensional array
  Body : Concatenate  NumInputs=3  Mode=Multidimensional array  ConcatenateDimension=2
  WheelFrontLeft : Concatenate  NumInputs=3  Mode=Multidimensional array  ConcatenateDimension=2
  WheelFrontRight : Concatenate  NumInputs=3  Mode=Multidimensional array  ConcatenateDimension=2
  WheelRearLeft : Concatenate  NumInputs=3  Mode=Multidimensional array  ConcatenateDimension=2
  WheelRearRight : Concatenate  NumInputs=3  Mode=Multidimensional array  ConcatenateDimension=2
  ConcatOut : Outport  VectorParamsAs1DForOutWhenUnconnected=off
  wires:
  BodyX/1 -> Body/1
  BodyZ/1 -> Body/3
  WheelFrontLeftX/1 -> WheelFrontLeft/1
  WheelFrontLeftZ/1 -> WheelFrontLeft/3
  WheelFrontLeftY/1 -> WheelFrontLeft/2
  BodyY/1 -> Body/2
  WheelFrontLeft/1 -> AllParts/2
  WheelRearRightX/1 -> WheelRearRight/1
  Body/1 -> AllParts/1
  WheelRearLeft/1 -> AllParts/4
  WheelFrontRight/1 -> AllParts/3
  WheelRearRightZ/1 -> WheelRearRight/3
  WheelFrontRightY/1 -> WheelFrontRight/2
  WheelFrontRightX/1 -> WheelFrontRight/1
  WheelRearRightY/1 -> WheelRearRight/2
  WheelRearLeftZ/1 -> WheelRearLeft/3
  AllParts/1 -> ConcatOut/1
  WheelRearLeftY/1 -> WheelRearLeft/2
  WheelRearRight/1 -> AllParts/5
  WheelRearLeftX/1 -> WheelRearLeft/1
  WheelFrontRightZ/1 -> WheelFrontRight/3

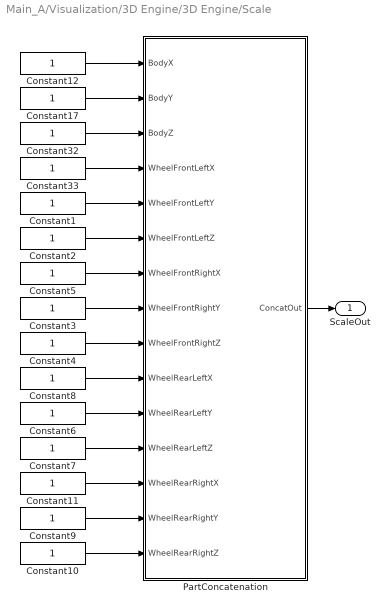
== system Main_A/Visualization/3D Engine/3D Engine/Scale ==
  Constant{1..12,17,32..33} (15 alike) : Constant  OutDataTypeStr=single
  PartConcatenation : Subsystem
  ScaleOut : Outport  VectorParamsAs1DForOutWhenUnconnected=off
  wires:
  Constant10/1 -> PartConcatenation/15(WheelRearRightZ)
  Constant9/1 -> PartConcatenation/14(WheelRearRightY)
  Constant11/1 -> PartConcatenation/13(WheelRearRightX)
  Constant7/1 -> PartConcatenation/12(WheelRearLeftZ)
  Constant6/1 -> PartConcatenation/11(WheelRearLeftY)
  Constant8/1 -> PartConcatenation/10(WheelRearLeftX)
  Constant4/1 -> PartConcatenation/9(WheelFrontRightZ)
  Constant3/1 -> PartConcatenation/8(WheelFrontRightY)
  Constant5/1 -> PartConcatenation/7(WheelFrontRightX)
  Constant2/1 -> PartConcatenation/6(WheelFrontLeftZ)
  Constant1/1 -> PartConcatenation/5(WheelFrontLeftY)
  Constant33/1 -> PartConcatenation/4(WheelFrontLeftX)
  Constant32/1 -> PartConcatenation/3(BodyZ)
  Constant17/1 -> PartConcatenation/2(BodyY)
  Constant12/1 -> PartConcatenation/1(BodyX)
  PartConcatenation/1(ConcatOut) -> ScaleOut/1

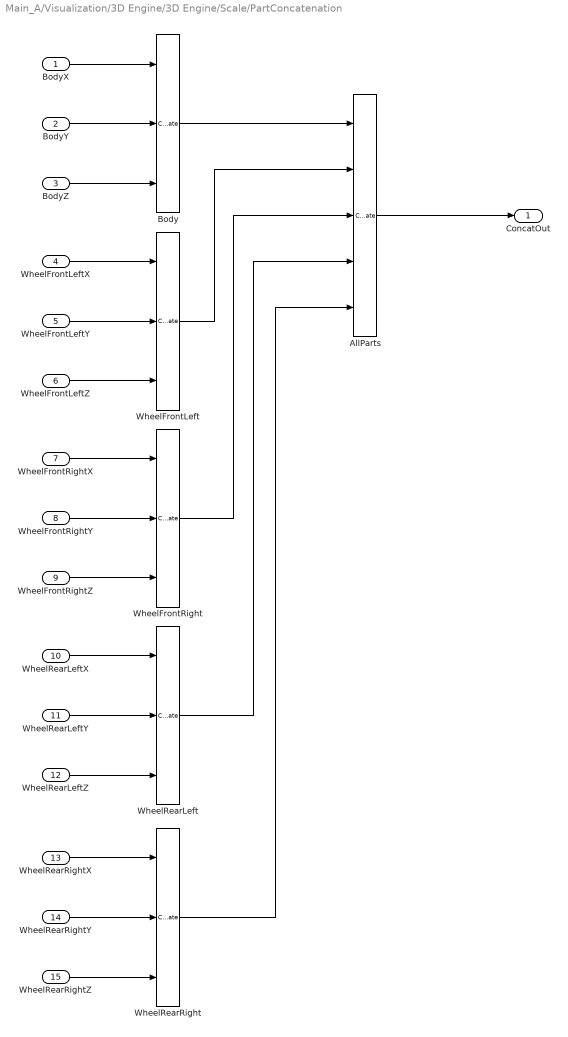
== system Main_A/Visualization/3D Engine/3D Engine/Scale/PartConcatenation ==
  BodyX : Inport
  BodyY : Inport  Port=2
  BodyZ : Inport  Port=3
  WheelFrontLeftX : Inport  Port=4
  WheelFrontLeftY : Inport  Port=5
  WheelFrontLeftZ : Inport  Port=6
  WheelFrontRightX : Inport  Port=7
  WheelFrontRightY : Inport  Port=8
  WheelFrontRightZ : Inport  Port=9
  WheelRearLeftX : Inport  Port=10
  WheelRearLeftY : Inport  Port=11
  WheelRearLeftZ : Inport  Port=12
  WheelRearRightX : Inport  Port=13
  WheelRearRightY : Inport  Port=14
  WheelRearRightZ : Inport  Port=15
  AllParts : Concatenate  NumInputs=5  Mode=Multidimensional array
  Body : Concatenate  NumInputs=3  Mode=Multidimensional array  ConcatenateDimension=2
  WheelFrontLeft : Concatenate  NumInputs=3  Mode=Multidimensional array  ConcatenateDimension=2
  WheelFrontRight : Concatenate  NumInputs=3  Mode=Multidimensional array  ConcatenateDimension=2
  WheelRearLeft : Concatenate  NumInputs=3  Mode=Multidimensional array  ConcatenateDimension=2
  WheelRearRight : Concatenate  NumInputs=3  Mode=Multidimensional array  ConcatenateDimension=2
  ConcatOut : Outport  VectorParamsAs1DForOutWhenUnconnected=off
  wires:
  BodyX/1 -> Body/1
  BodyZ/1 -> Body/3
  WheelFrontLeftX/1 -> WheelFrontLeft/1
  WheelFrontLeftZ/1 -> WheelFrontLeft/3
  WheelFrontLeftY/1 -> WheelFrontLeft/2
  BodyY/1 -> Body/2
  WheelFrontLeft/1 -> AllParts/2
  WheelRearRightX/1 -> WheelRearRight/1
  Body/1 -> AllParts/1
  WheelRearLeft/1 -> AllParts/4
  WheelFrontRight/1 -> AllParts/3
  WheelRearRightZ/1 -> WheelRearRight/3
  WheelFrontRightY/1 -> WheelFrontRight/2
  WheelFrontRightX/1 -> WheelFrontRight/1
  WheelRearRightY/1 -> WheelRearRight/2
  WheelRearLeftZ/1 -> WheelRearLeft/3
  AllParts/1 -> ConcatOut/1
  WheelRearLeftY/1 -> WheelRearLeft/2
  WheelRearRight/1 -> AllParts/5
  WheelRearLeftX/1 -> WheelRearLeft/1
  WheelFrontRightZ/1 -> WheelFrontRight/3

== matlab function Main_A/Environment/EnhancedSplitMu/SplitMu Function ==
  data: VehDim input; X input; mu_FL output; Y input; psi input; SplitMu input; SplitLine input; mu_FR output; mu_RL output; mu_RR output; XorY input
function [mu_FL,mu_FR,mu_RL,mu_RR] = fcn(VehDim,X,Y,psi,SplitMu,SplitLine,XorY)

% Right-hand rule ******************************************************* %
%   X                                                                     %
%   |             - X-axis aligns with vehicle's longitudinal axis        %
%   |             - Z-axis points downwards                               %
%   |_ _ _ _ Y                                                            %
% *********************************************************************** %

% Vehicle dimensions
TW2   = VehDim(1)/2;   % Track width divided by 2
CG2FA = VehDim(2);     % Distance from CG to front axle
CG2RA = VehDim(3);     % Distance from CG to rear axle

% Inertial frame coordinates
CG = [X; Y];           % Location of the vehicle in the inertial frame

% Vehicle's body frame coordinates [x; y]
CG2FL = [ CG2FA; -TW2];
CG2FR = [ CG2FA;  TW2];
CG2RL = [-CG2RA; -TW2];
CG2RR = [-CG2RA;  TW2];

% Rotation matrix
R = [cos(psi), -sin(psi);...
     sin(psi),  cos(psi)];

% Coordinate transformation of body frame to inertial frame
O_FL = R * CG2FL + CG;
O_FR = R * CG2FR + CG;
O_RL = R * CG2RL + CG;
O_RR = R * CG2RR + CG;

% Mu selection for each wheel based on the "surface" they are on.
% Each vector follows the definition [FL; FR; RL; RR]
if XorY == true
    temp = 1;
else
    temp = 2;
end
O_split = [O_FL(temp); O_FR(temp); O_RL(temp); O_RR(temp)];
Mu   = zeros(4,1);

for i = 1:4
    if O_split(i) < SplitLine
        Mu(i) = SplitMu(1);
    else
        Mu(i) = SplitMu(2);
    end
end

mu_FL = Mu(1);
mu_FR = Mu(2);
mu_RL = Mu(3);
mu_RR = Mu(4);

end
